simulink model "Two_Channel_PP_Teleoperation"  (R2022b)
settings: Solver=VariableStepAuto  StartTime=0.0  StopTime=5  RelTol=1e-3
values from neighbouring files (symbols this model uses):
  A = 200    [parameters.m]
  Be = 100    [parameters.m]
  Bh = 1    [parameters.m]
  Bm = 20*0.8    (= 16)    [parameters.m]
  Bs = 4*Bm    (= 64)    [parameters.m]
  Dh = 20*0.8    (= 16)    [parameters.m]
  Dm = 0.3    [parameters.m]
  Ds = 1.2    [parameters.m]
  Fc = 1    [parameters.m]
  Flp = 0.5    [parameters.m]
  Jh = 1    [parameters.m]
  Ke = 200    [parameters.m]
  Km = 10*1    (= 10)    [parameters.m]
  Ks = 4*Km    (= 40)    [parameters.m]
  Mm = 0.5    [parameters.m]
  Ms = 2    [parameters.m]
  Ph = 10*1    (= 10)    [parameters.m]
  xe = 15    [parameters.m]
settings Model: Creator=uzair  LastModifiedBy=uzair

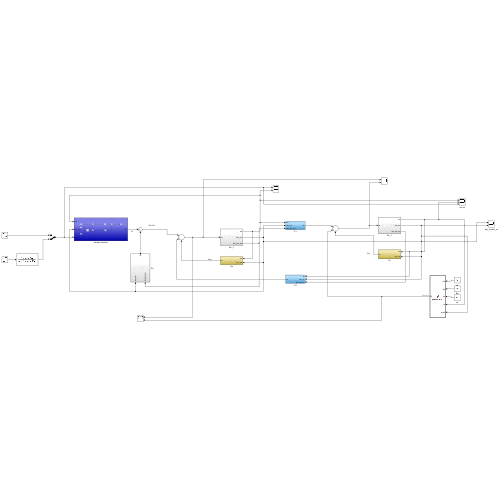
[thumbnail: Simulink's stored preview of the top-level diagram]
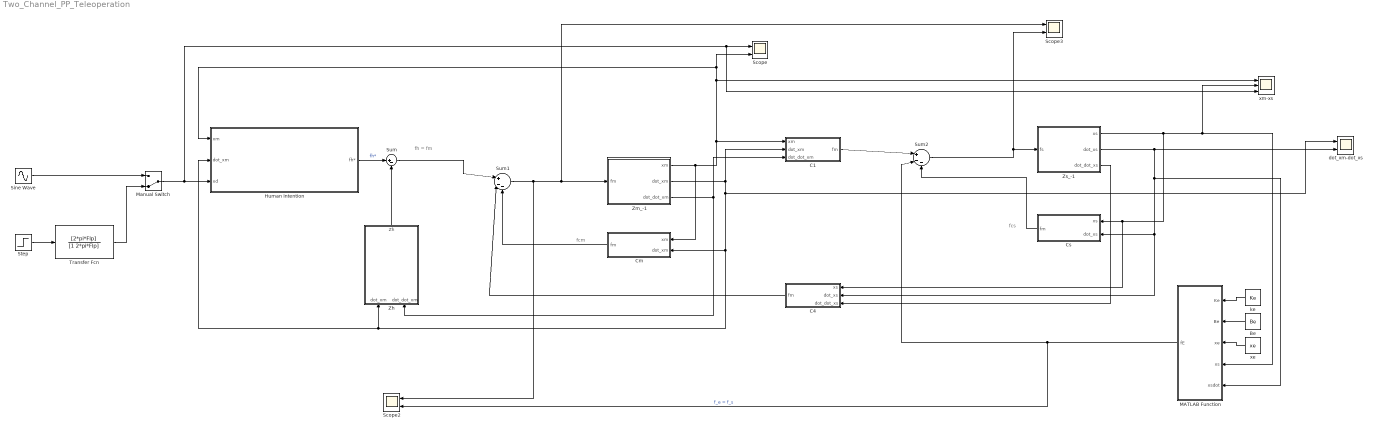
== system Two_Channel_PP_Teleoperation ==
  note: fcs
  note: fcm
  note: fh = fm
  Be : Constant  Value=Be
  C1 : Subsystem
  C4 : Subsystem
  Cm : Subsystem
  Cs : Subsystem
  Human Intention : Subsystem
  MATLAB Function : MATLAB Function  TreatAsAtomicUnit=on
  Manual Switch : ManualSwitch  CurrentSetting=0
  Scope : Scope  NumInputPorts=2
  Scope2 : Scope  NumInputPorts=2
  Scope3 : Scope  NumInputPorts=2
  Sine Wave : Sin  Amplitude=A  Frequency=2*pi*Fc  SampleTime=0
  Step : Step  Time=0.5  After=A  SampleTime=0
  Sum : Sum  Inputs=|+-
  Sum1 : Sum  Inputs=|+--
  Sum2 : Sum  Inputs=|+--
  Transfer Fcn : TransferFcn  Numerator=[2*pi*Flp]  Denominator=[1 2*pi*Flp]
  Zh : Subsystem
  Zm_-1 : Subsystem
  Zs_-1 : Subsystem
  dot_xm-dot_xs : Scope  NumInputPorts=2
  ke : Constant  Value=Ke
  xe : Constant  Value=xe
  xm-xs : Scope  NumInputPorts=3
  wires:
  Sine Wave/1 -> Manual Switch/1
  Step/1 -> Transfer Fcn/1
  Transfer Fcn/1 -> Manual Switch/2
  Manual Switch/1 -> xm-xs/3, Scope/1, Human Intention/3(xd)
  Human Intention/1(fh*) -> Sum/1  "fh*"
  Zh/1(Zh) -> Sum/2
  Sum/1 -> Sum1/1
  Sum1/1 -> Scope2/1, Scope3/1, Zm_-1/1(fm)
  Zm_-1/3(dot_dot_xm) -> C1/3(dot_dot_xm), Zh/2(dot_dot_xm)
  Zm_-1/2(dot_xm) -> C1/2(dot_xm), dot_xm-dot_xs/1, Human Intention/2(dot_xm), Zh/1(dot_xm), Cm/2(dot_xm)
  Cm/1(fm) -> Sum1/3
  C4/1(fm) -> Sum1/2
  Sum2/1 -> Scope3/2, Zs_-1/1(fs)
  Cs/1(fm) -> Sum2/3
  Zs_-1/1(xs) -> C4/1(xs), Cs/1(xs), xm-xs/2, MATLAB Function/4(xs)
  Zs_-1/2(dot_xs) -> dot_xm-dot_xs/2, MATLAB Function/5(xsdot), C4/2(dot_xs), Cs/2(dot_xs)
  xe/1 -> MATLAB Function/3(xe)
  Be/1 -> MATLAB Function/2(Be)
  ke/1 -> MATLAB Function/1(Ke)
  MATLAB Function/1(fE) -> Sum2/2, Scope2/2  "f_e = f_s"
  Zs_-1/3(dot_dot_xs) -> C4/3(dot_dot_xs)
  Zm_-1/1(xm) -> Cm/1(xm), Scope/2, Human Intention/1(xm), xm-xs/1, C1/1(xm)
  C1/1(fm) -> Sum2/1

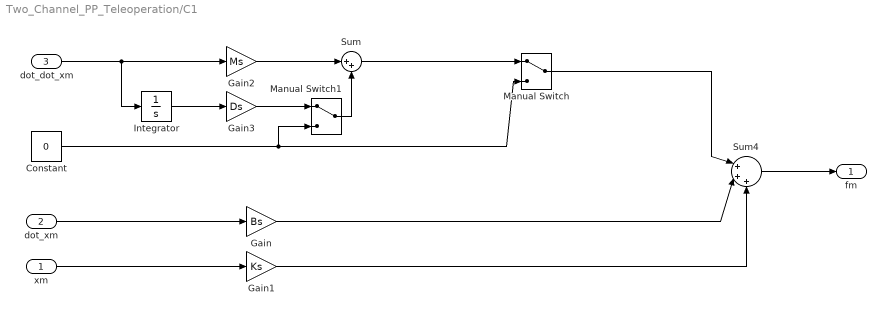
== system Two_Channel_PP_Teleoperation/C1 ==
  xm : Inport
  dot_xm : Inport  Port=2
  dot_dot_xm : Inport  Port=3
  Constant : Constant  Value=0
  Gain : Gain  Gain=Bs
  Gain1 : Gain  Gain=Ks
  Gain2 : Gain  Gain=Ms
  Gain3 : Gain  Gain=Ds
  Integrator : Integrator
  Manual Switch : ManualSwitch
  Manual Switch1 : ManualSwitch
  Sum : Sum  Inputs=|++
  Sum4 : Sum  Inputs=|+++
  fm : Outport
  wires:
  dot_xm/1 -> Gain/1
  Gain/1 -> Sum4/2
  xm/1 -> Gain1/1
  Sum4/1 -> fm/1
  Gain1/1 -> Sum4/3
  Sum/1 -> Manual Switch/1
  Manual Switch/1 -> Sum4/1
  Constant/1 -> Manual Switch1/2, Manual Switch/2
  dot_dot_xm/1 -> Integrator/1, Gain2/1
  Integrator/1 -> Gain3/1
  Gain2/1 -> Sum/1
  Gain3/1 -> Manual Switch1/1
  Manual Switch1/1 -> Sum/2

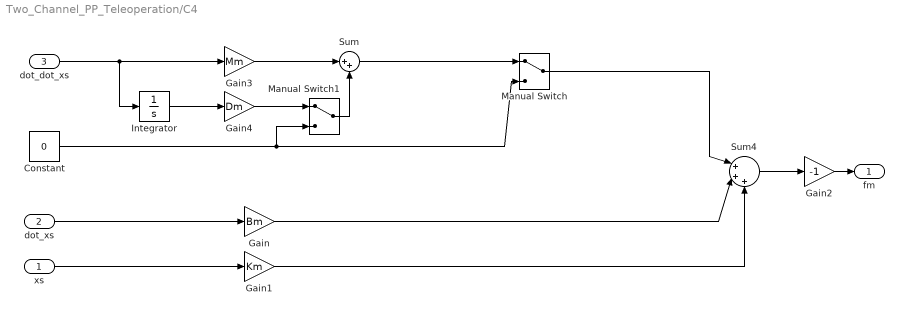
== system Two_Channel_PP_Teleoperation/C4 ==
  xs : Inport
  dot_xs : Inport  Port=2
  dot_dot_xs : Inport  Port=3
  Constant : Constant  Value=0
  Gain : Gain  Gain=Bm
  Gain1 : Gain  Gain=Km
  Gain2 : Gain  Gain=-1
  Gain3 : Gain  Gain=Mm
  Gain4 : Gain  Gain=Dm
  Integrator : Integrator
  Manual Switch : ManualSwitch
  Manual Switch1 : ManualSwitch
  Sum : Sum  Inputs=|++
  Sum4 : Sum  Inputs=|+++
  fm : Outport
  wires:
  Gain2/1 -> fm/1
  Sum/1 -> Manual Switch/1
  Gain3/1 -> Sum/1
  Manual Switch1/1 -> Sum/2
  Gain/1 -> Sum4/2
  Constant/1 -> Manual Switch1/2, Manual Switch/2
  Gain1/1 -> Sum4/3
  xs/1 -> Gain1/1
  Manual Switch/1 -> Sum4/1
  dot_xs/1 -> Gain/1
  dot_dot_xs/1 -> Integrator/1, Gain3/1
  Integrator/1 -> Gain4/1
  Gain4/1 -> Manual Switch1/1
  Sum4/1 -> Gain2/1

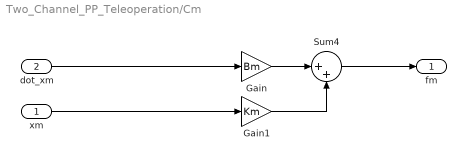
== system Two_Channel_PP_Teleoperation/Cm ==
  xm : Inport
  dot_xm : Inport  Port=2
  Gain : Gain  Gain=Bm
  Gain1 : Gain  Gain=Km
  Sum4 : Sum  Inputs=|++
  fm : Outport
  wires:
  Sum4/1 -> fm/1
  xm/1 -> Gain1/1
  Gain/1 -> Sum4/1
  Gain1/1 -> Sum4/2
  dot_xm/1 -> Gain/1

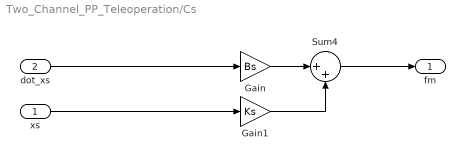
== system Two_Channel_PP_Teleoperation/Cs ==
  xs : Inport
  dot_xs : Inport  Port=2
  Gain : Gain  Gain=Bs
  Gain1 : Gain  Gain=Ks
  Sum4 : Sum  Inputs=|++
  fm : Outport
  wires:
  Sum4/1 -> fm/1
  xs/1 -> Gain1/1
  Gain/1 -> Sum4/1
  Gain1/1 -> Sum4/2
  dot_xs/1 -> Gain/1

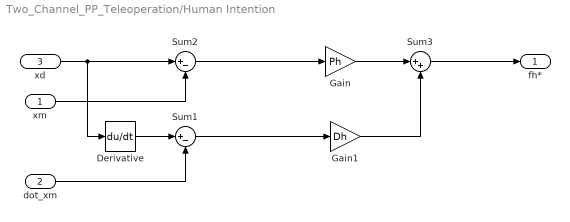
== system Two_Channel_PP_Teleoperation/Human Intention ==
  xm : Inport
  dot_xm : Inport  Port=2
  xd : Inport  Port=3
  Derivative : Derivative
  Gain : Gain  Gain=Ph
  Gain1 : Gain  Gain=Dh
  Sum1 : Sum  Inputs=|+-
  Sum2 : Sum  Inputs=|+-
  Sum3 : Sum  Inputs=|++
  fh* : Outport
  wires:
  xm/1 -> Sum2/2
  dot_xm/1 -> Sum1/2
  Sum2/1 -> Gain/1
  Sum1/1 -> Gain1/1
  Gain1/1 -> Sum3/2
  Gain/1 -> Sum3/1
  Sum3/1 -> fh*/1
  xd/1 -> Derivative/1, Sum2/1
  Derivative/1 -> Sum1/1

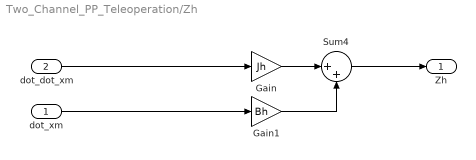
== system Two_Channel_PP_Teleoperation/Zh ==
  dot_xm : Inport
  dot_dot_xm : Inport  Port=2
  Gain : Gain  Gain=Jh
  Gain1 : Gain  Gain=Bh
  Sum4 : Sum  Inputs=|++
  Zh : Outport
  wires:
  dot_dot_xm/1 -> Gain/1
  Gain1/1 -> Sum4/2
  Gain/1 -> Sum4/1
  Sum4/1 -> Zh/1
  dot_xm/1 -> Gain1/1

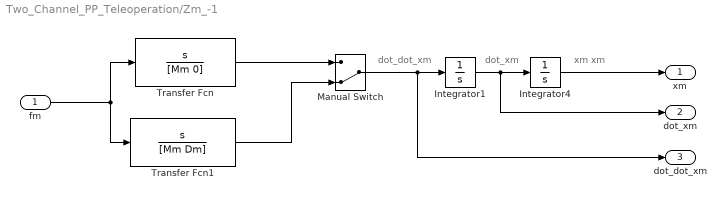
== system Two_Channel_PP_Teleoperation/Zm_-1 ==
  note: dot_dot_xm
  note: dot_xm
  note: xm
      | xm
  fm : Inport
  Integrator1 : Integrator
  Integrator4 : Integrator
  Manual Switch : ManualSwitch  CurrentSetting=0
  Transfer Fcn : TransferFcn  Numerator=[1 0]  Denominator=[Mm 0]
  Transfer Fcn1 : TransferFcn  Numerator=[1 0]  Denominator=[Mm Dm]
  xm : Outport
  dot_xm : Outport  Port=2
  dot_dot_xm : Outport  Port=3
  wires:
  Manual Switch/1 -> dot_dot_xm/1, Integrator1/1
  Integrator4/1 -> xm/1
  Integrator1/1 -> dot_xm/1, Integrator4/1
  fm/1 -> Transfer Fcn/1, Transfer Fcn1/1
  Transfer Fcn/1 -> Manual Switch/1
  Transfer Fcn1/1 -> Manual Switch/2

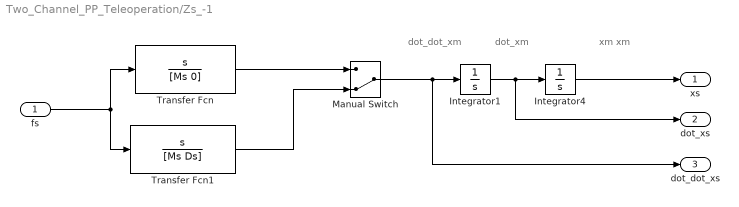
== system Two_Channel_PP_Teleoperation/Zs_-1 ==
  note: dot_dot_xm
  note: dot_xm
  note: xm
      | xm
  fs : Inport
  Integrator1 : Integrator
  Integrator4 : Integrator
  Manual Switch : ManualSwitch  CurrentSetting=0
  Transfer Fcn : TransferFcn  Numerator=[1 0]  Denominator=[Ms 0]
  Transfer Fcn1 : TransferFcn  Numerator=[1 0]  Denominator=[Ms Ds]
  xs : Outport
  dot_xs : Outport  Port=2
  dot_dot_xs : Outport  Port=3
  wires:
  Manual Switch/1 -> dot_dot_xs/1, Integrator1/1
  Integrator4/1 -> xs/1
  Integrator1/1 -> dot_xs/1, Integrator4/1
  fs/1 -> Transfer Fcn/1, Transfer Fcn1/1
  Transfer Fcn/1 -> Manual Switch/1
  Transfer Fcn1/1 -> Manual Switch/2

== matlab function Two_Channel_PP_Teleoperation/MATLAB Function ==
  data: Ke input; fE output; Be input; xe input; xs input; xsdot input
function fE = environment(Ke, Be, xe, xs, xsdot)
    if xs > xe
        fE = Ke * (xs - xe) + Be * xsdot; % Plot both contributions Ke and Be
    else
        fE = 0;
    end
end
